simulink model "Deadlock"  (R2025a)
settings: Solver=FixedStepDiscrete  StartTime=0.0  StopTime=10.0  FixedStep=.1  RelTol=1e-3
undefined symbols (not defined in the file or in its folder): DiscIntNeverNeededParam
libraries: simulink x2
settings Model: Creator=nirmay  LastModifiedBy=nirmay

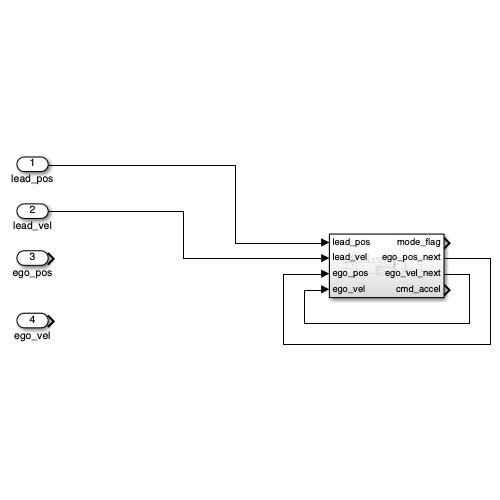
[thumbnail: Simulink's stored preview of the top-level diagram]
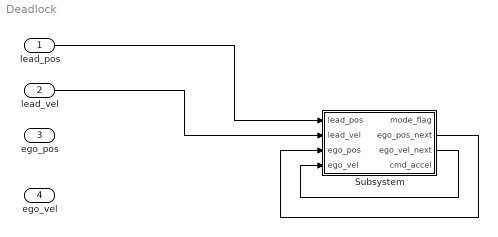
== system Deadlock ==
  lead_pos : Inport
  lead_vel : Inport  Port=2
  ego_pos : Inport  Port=3
  ego_vel : Inport  Port=4
  Subsystem : Subsystem
  wires:
  lead_pos/1 -> Subsystem/1(lead_pos)
  lead_vel/1 -> Subsystem/2(lead_vel)
  Subsystem/2(ego_pos_next) -> Subsystem/3(ego_pos)
  Subsystem/3(ego_vel_next) -> Subsystem/4(ego_vel)

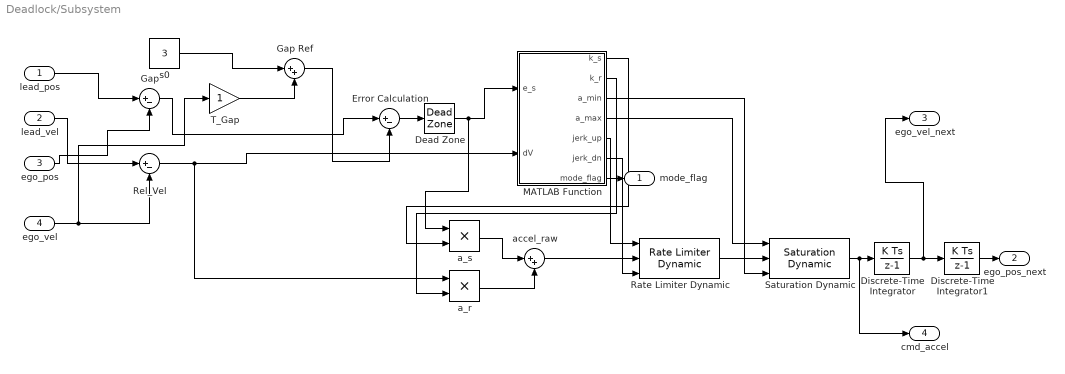
== system Deadlock/Subsystem ==
  lead_pos : Inport
  lead_vel : Inport  Port=2
  ego_pos : Inport  Port=3
  ego_vel : Inport  Port=4
  Dead Zone : DeadZone  LowerValue=-1  UpperValue=1
  Discrete-Time Integrator : DiscreteIntegrator  SampleTime=-1  ICPrevOutput=DiscIntNeverNeededParam  ICPrevScaledInput=DiscIntNeverNeededParam
  Discrete-Time Integrator1 : DiscreteIntegrator  SampleTime=-1  ICPrevOutput=DiscIntNeverNeededParam  ICPrevScaledInput=DiscIntNeverNeededParam
  Error Calculation : Sum  Inputs=|+-
  Gap : Sum  Inputs=|+-
  Gap Ref : Sum  Inputs=|++
  MATLAB Function : MATLAB Function  TreatAsAtomicUnit=on
  Rate Limiter Dynamic : simulink/Discontinuities/Rate Limiter Dynamic
  Rel_Vel : Sum  Inputs=|+-
  Saturation Dynamic : simulink/Discontinuities/Saturation Dynamic  OutMin=[]  OutMax=[]  OutDataTypeStr=Inherit: Same as second input  OutDataType=fixdt(1, 16)  OutScaling=2^-10  DoSatur=off
  T_Gap : Gain
  a_r : Product
  a_s : Product
  accel_raw : Sum  Inputs=|++
  s0 : Constant  Value=3
  mode_flag : Outport
  ego_pos_next : Outport  Port=2
  ego_vel_next : Outport  Port=3
  cmd_accel : Outport  Port=4
  wires:
  MATLAB Function/5(jerk_up) -> Rate Limiter Dynamic/1
  Saturation Dynamic/1 -> cmd_accel/1, Discrete-Time Integrator/1
  a_r/1 -> accel_raw/2
  Discrete-Time Integrator1/1 -> ego_pos_next/1
  ego_pos/1 -> Gap/2
  MATLAB Function/3(a_min) -> Saturation Dynamic/3
  MATLAB Function/6(jerk_dn) -> Rate Limiter Dynamic/3
  MATLAB Function/2(k_r) -> a_r/2
  Error Calculation/1 -> Dead Zone/1
  MATLAB Function/1(k_s) -> a_s/2
  Rel_Vel/1 -> a_r/1, MATLAB Function/2(dV)
  ego_vel/1 -> T_Gap/1, Rel_Vel/2
  lead_pos/1 -> Gap/1
  Discrete-Time Integrator/1 -> ego_vel_next/1, Discrete-Time Integrator1/1
  MATLAB Function/4(a_max) -> Saturation Dynamic/1
  Gap/1 -> Error Calculation/1
  Gap Ref/1 -> Error Calculation/2
  T_Gap/1 -> Gap Ref/2
  a_s/1 -> accel_raw/1
  Rate Limiter Dynamic/1 -> Saturation Dynamic/2
  MATLAB Function/7(mode_flag) -> mode_flag/1
  accel_raw/1 -> Rate Limiter Dynamic/2
  s0/1 -> Gap Ref/1
  Dead Zone/1 -> a_s/1, MATLAB Function/1(e_s)
  lead_vel/1 -> Rel_Vel/1

== matlab function Deadlock/Subsystem/MATLAB Function ==
  data: e_s input; k_s output; dV input; k_r output; a_min output; a_max output; jerk_up output; jerk_dn output; mode_flag output
function [k_s,k_r,a_min,a_max,jerk_up,jerk_dn,mode_flag] = mode_manager(e_s,dV)
% Default (Normal)
k_s=0.20; k_r=0.60;
a_min=-3.0; a_max=2.0;
jerk_up=2.0; jerk_dn=-2.0;
mode_flag=1; % 1=Normal,2=Protect,3=Pursue

% Thresholds
e_hi=5; e_lo=3; dV_hi=1;

% Protect (too close or closing fast)
if (e_s < -e_lo) || (dV < -dV_hi)
    k_s=0.35; k_r=0.40;
    a_min=-3.5; jerk_dn=-2.5;
    mode_flag=2;
elseif (e_s > e_hi && dV > 0)
    % Pursue (gap growing)
    k_s=0.15; k_r=0.75;
    mode_flag=3;
end
end
